simulink model "Movimento_horizontal"  (R2019b)
settings: Solver=VariableStepAuto  StartTime=0.0  StopTime=10000  RelTol=1e-3
undefined symbols (not defined in the file): rho
libraries: simulink x1
settings Model: Creator=Ethianne  LastModifiedBy=Ethianne

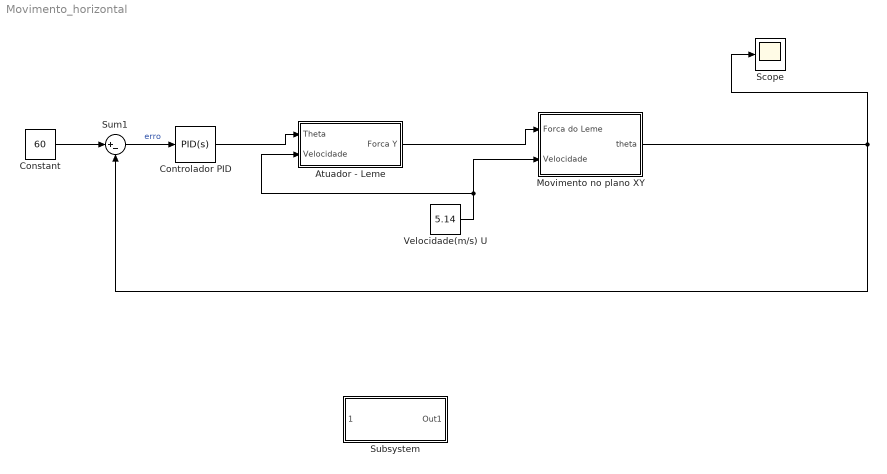
== system Movimento_horizontal ==
  Atuador - Leme : Subsystem
  Constant : Constant  Value=60
  "Controlador PID " : simulink/Continuous/PID Controller  Controller=PID  Form=Parallel  TimeDomain=Continuous-time  SampleTime=-1  IntegratorMethod=Forward Euler  FilterMethod=Forward Euler  ControllerParametersSource=internal  P=0.6600732151374  I=0.0236056860866178  D=4.02588249963261  UseFilter=on  N=6.15024402255971  TunerSelectOption=Transfer Function Based (PID Tuner App)  InitialConditionSource=internal  InitialConditionForIntegrator=0  InitialConditionForFilter=0  DifferentiatorICPrevScaledInput=0  ExternalReset=none  TrackingMode=off  Kt=1  LimitOutput=off  UpperSaturationLimit=inf  LowerSaturationLimit=-inf  LinearizeAsGain=on  AntiWindupMode=none  Kb=1  POutMin=[]  POutMax=[]  IOutMin=[]  IOutMax=[]  DOutMin=[]  DOutMax=[]  NOutMin=[]  NOutMax=[]  SumOutMin=[]  SumOutMax=[]  SaturationOutMin=[]  SaturationOutMax=[]  PParamMin=[]  PParamMax=[]  IParamMin=[]  IParamMax=[]  DParamMin=[]  DParamMax=[]  NParamMin=[]  NParamMax=[]  KbParamMin=[]  KbParamMax=[]  KtParamMin=[]  KtParamMax=[]  KbOutMin=[]  KbOutMax=[]  KtOutMin=[]  KtOutMax=[]  IntegratorOutMin=[]  IntegratorOutMax=[]  FilterOutMin=[]  FilterOutMax=[]  SumI1OutMin=[]  SumI1OutMax=[]  SumI2OutMin=[]  SumI2OutMax=[]  SumI3OutMin=[]  SumI3OutMax=[]  SumI4OutMin=[]  SumI4OutMax=[]  SumDOutMin=[]  SumDOutMax=[]  DifferentiatorOutMin=[]  DifferentiatorOutMax=[]  FilterDiffOutCoefMin=[]  FilterDiffOutCoefMax=[]  ReciprocalOutMin=[]  ReciprocalOutMax=[]  SumDenOutMin=[]  SumDenOutMax=[]  SumNumOutMin=[]  SumNumOutMax=[]  DivideOutMin=[]  DivideOutMax=[]  IntegratorContinuousStateAttributes=''  IntegratorStateMustResolveToSignalObject=off  IntegratorRTWStateStorageClass=Auto  FilterContinuousStateAttributes=''  FilterStateMustResolveToSignalObject=off  FilterRTWStateStorageClass=Auto  ParallelPVariant=InternalParameters  IdealPVariant=Disabled  IVariant=InternalParameters  DVariant=InternalParameters  IntegratorVariant=Continuous  SatVariant=Disabled  AWVariant=Passthrough  PCopyVariant=Disabled  TRVariant=Disabled  FdbkBlocksVariant=Forward  IdealPFdbkVariant=Disabled  SatFdbkVariant=Disabled  DerivativeFilterVariant=ContFilter  NVariant=InternalParameters  NCopyVariant=Disabled  FilterICVariant=InternalICsFilter  IntegratorICVariant=InternalICs  ExternalResetVariant=Disabled  TRSumVariant=Passthrough  SumFdbkVariant=Disabled  SumVariant=Sum_PID
  Movimento no plano XY : Subsystem
  Scope : Scope
  Subsystem : Subsystem
  Sum1 : Sum  Inputs=|+-
  Velocidade(m/s) U : Constant  Value=5.14
  wires:
  Movimento no plano XY/1(theta) -> Scope/1, Sum1/2
  "Controlador PID "/1 -> Atuador - Leme/1("Theta ")
  Sum1/1 -> "Controlador PID "/1  "erro"
  Constant/1 -> Sum1/1
  Atuador - Leme/1(Forca Y) -> Movimento no plano XY/1("Forca do Leme ")
  Velocidade(m/s) U/1 -> Movimento no plano XY/2("Velocidade "), Atuador - Leme/2("Velocidade ")

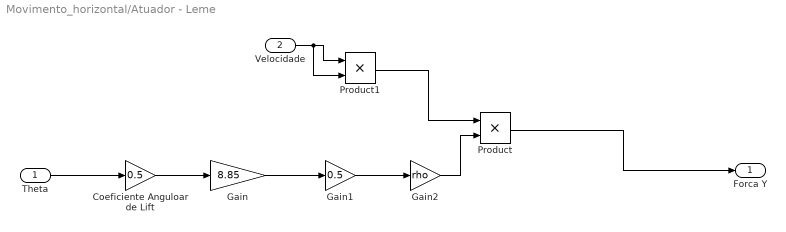
== system Movimento_horizontal/Atuador - Leme ==
  "Theta " : Inport
  "Velocidade " : Inport  Port=2
  Coeficiente Anguloar de Lift : Gain  Gain=0.5
  Gain : Gain  Gain=8.85
  Gain1 : Gain  Gain=0.5
  Gain2 : Gain  Gain=rho
  Product : Product
  Product1 : Product
  Forca Y : Outport
  wires:
  "Theta "/1 -> Coeficiente Anguloar de Lift/1
  Gain1/1 -> Gain2/1
  Coeficiente Anguloar de Lift/1 -> Gain/1
  Gain/1 -> Gain1/1
  Gain2/1 -> Product/2
  "Velocidade "/1 -> Product1/2, Product1/1
  Product1/1 -> Product/1
  Product/1 -> Forca Y/1

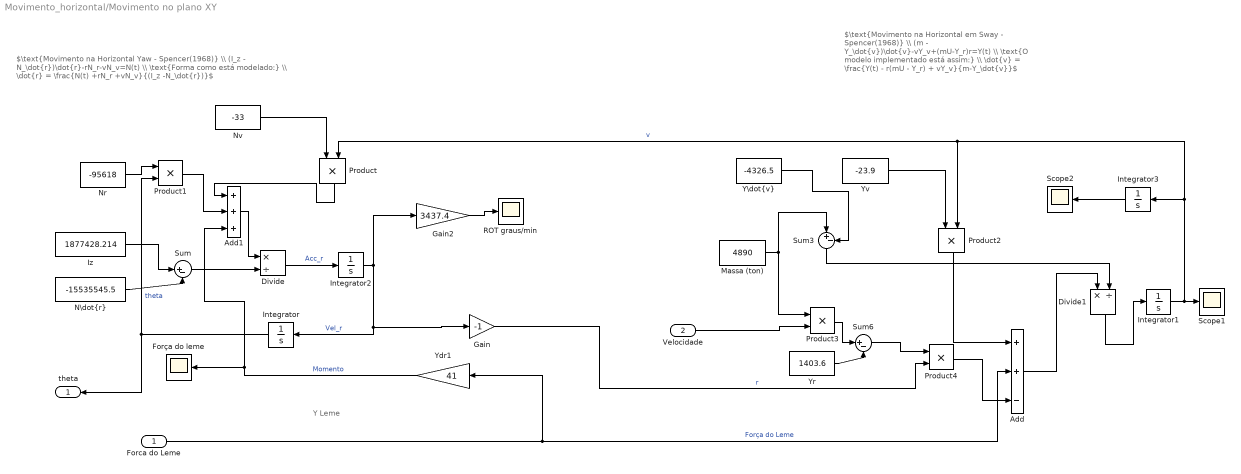
== system Movimento_horizontal/Movimento no plano XY ==
  note: Y Leme
  note: $\text{Movimento na Horizontal Yaw - Spencer(1968)} \\ (I_z - N_\dot{r})\dot{r}-rN_r-vN_v=N(t) \\ \text{Forma como está modelado:} \\ \dot{r} = \frac{N(t) +rN_r +vN_v}{(I_z -N_\dot{r})}$
  note: $\text{Movimento na Horizontal em Sway - Spencer(1968)} \\ (m - Y_\dot{v})\dot{v}-vY_v+(mU-Y_r)r=Y(t) \\ \text{O modelo implementado está assim:} \\ \dot{v} = \frac{Y(t) - r(mU - Y_r) + vY_v}{m-Y_\dot{v}}$
  "Forca do Leme " : Inport
  "Velocidade " : Inport  Port=2
  Add : Sum  Inputs=++-
  Add1 : Sum  Inputs=+++
  Divide : Product  Inputs=*/
  Divide1 : Product  Inputs=*/
  Força do leme : Scope
  Gain : Gain  Gain=-1
  Gain2 : Gain  Gain=3437.4
  Integrator{,1..3} (4 alike) : Integrator
  Iz : Constant  Value=1877428.214
  Massa (ton) : Constant  Value=4890
  "N\\dot{r}" : Constant  Value=-15535545.5
  Nr : Constant  Value=-95618
  "Nv " : Constant  Value=-33
  Product{,1..4} (5 alike) : Product
  ROT graus/min : Scope
  Scope1 : Scope
  Scope2 : Scope
  Sum : Sum  Inputs=|+-
  Sum3 : Sum  Inputs=|+-
  Sum6 : Sum  Inputs=|+-
  "Y\\dot{v}" : Constant  Value=-4326.5
  Ydr1 : Gain  Gain=41
  Yr : Constant  Value=1403.6
  Yv : Constant  Value=-23.9
  theta : Outport
  wires:
  Massa (ton)/1 -> Product3/1, Sum3/1
  Integrator1/1 -> Product2/2, Product/2, Integrator3/1, Scope1/1  "v"
  Sum/1 -> Divide/2
  Divide/1 -> Integrator2/1  "Acc_r"
  "Forca do Leme "/1 -> Add/2, Ydr1/1  "Força do Leme"
  Add/1 -> Divide1/1
  Integrator2/1 -> Gain/1, Integrator/1, Gain2/1  "Vel_r"
  Nr/1 -> Product1/1
  Product/1 -> Add1/1
  Yr/1 -> Sum6/2
  Yv/1 -> Product2/1
  "Nv "/1 -> Product/1
  Divide1/1 -> Integrator1/1
  Iz/1 -> Sum/1
  Add1/1 -> Divide/1
  Gain/1 -> Product4/2  "r"
  Sum6/1 -> Product4/1
  Product1/1 -> Add1/2
  "Y\\dot{v}"/1 -> Sum3/2
  Ydr1/1 -> Add1/3, Força do leme/1  "Momento"
  Product3/1 -> Sum6/1
  "Velocidade "/1 -> Product3/2
  Integrator3/1 -> Scope2/1
  "N\\dot{r}"/1 -> Sum/2
  Gain2/1 -> ROT graus/min/1
  Sum3/1 -> Divide1/2
  Product4/1 -> Add/3
  Product2/1 -> Add/1
  Integrator/1 -> Product1/2, theta/1  "theta"

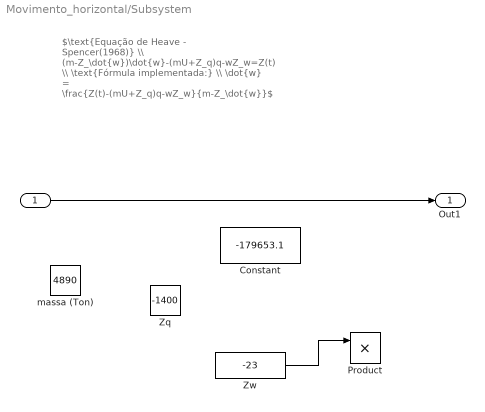
== system Movimento_horizontal/Subsystem ==
  note: $\text{Equação de Heave - Spencer(1968)} \\ (m-Z_\dot{w})\dot{w}-(mU+Z_q)q-wZ_w=Z(t) \\ \text{Fórmula implementada:} \\ \dot{w} = \frac{Z(t)-(mU+Z_q)q-wZ_w}{m-Z_\dot{w}}$
  " " : Inport
  Constant : Constant  Value=-179653.1
  Product : Product
  Zq : Constant  Value=-1400
  Zw : Constant  Value=-23
  massa (Ton) : Constant  Value=4890
  Out1 : Outport
  wires:
  " "/1 -> Out1/1
  Zw/1 -> Product/1
